simulink model "deedemo1"  (Simulink 3.00)
settings: Solver=ode45  SolverMode=SingleTasking  StartTime=0.0  StopTime=999999  RelTol=1e-3  AbsTol=1e-6
settings Model: SaveTime=off  SaveOutput=off  Creator=sanjai  LastModifiedBy=sanjai

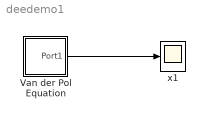
== system deedemo1 ==
  Van der Pol Equation : Subsystem
      settings: OpenFcn=diffeqed
      mask Type: Differential Equation Editor (DEE)
      mask Display: disp('vdp')
  x1 : Scope
      settings: TickLabels=on  TimeRange=20.000000  YMin=-3  YMax=3  SaveToWorkspace=off  SaveName=ScopeData  DataFormat=Matrix
  wires:
  Van der Pol Equation/1(Port1) -> x1/1

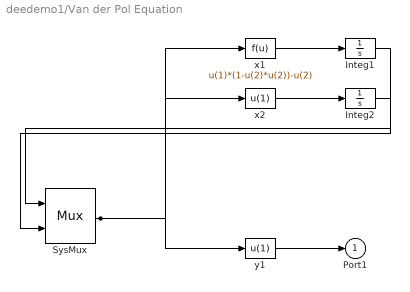
== system deedemo1/Van der Pol Equation ==
  Integ1 : Integrator  ExternalReset=none  InitialConditionSource=internal  InitialCondition=1  LimitOutput=off  UpperSaturationLimit=inf  LowerSaturationLimit=-inf  ShowSaturationPort=off  ShowStatePort=off  AbsoluteTolerance=auto
  Integ2 : Integrator  ExternalReset=none  InitialConditionSource=internal  InitialCondition=1  LimitOutput=off  UpperSaturationLimit=inf  LowerSaturationLimit=-inf  ShowSaturationPort=off  ShowStatePort=off  AbsoluteTolerance=auto
  SysMux : Mux  Inputs=2
      settings: DisplayOption=none
  x1 : Fcn  Expr=u(1)*(1-u(2)*u(2))-u(2)
  x2 : Fcn  Expr=u(1)
  y1 : Fcn  Expr=u(1)
  Port1 : Outport  Port=1  InitialOutput=0
  wires:
  y1/1 -> Port1/1
  SysMux/1 -> y1/1, x2/1, x1/1
  Integ2/1 -> SysMux/2
  x2/1 -> Integ2/1
  Integ1/1 -> SysMux/1
  x1/1 -> Integ1/1
